simulink model "test_MPC_var2"  (R2025b)
settings: Solver=VariableStepAuto  StartTime=0.0  StopTime=20  RelTol=1e-3
undefined symbols (not defined in the file): imp_amp_d, imp_dur_d, stp_amp_u, stp_tim_u
libraries: cstblocks x4, mpclib x1
settings Model: Creator=USER  LastModifiedBy=francesco
settings SolverCC: AlgebraicLoopSolver=TrustRegion
settings DebuggingCC: AlgebraicLoopMsg=none  UnconnectedInputMsg=warning  UnconnectedLineMsg=warning
settings ModelReferenceCC: EnableRefExpFcnMdlSchedulingChecks=on
settings RTWCC: GPUComputeCapability=3.5  DLArmComputeVersion=19.05

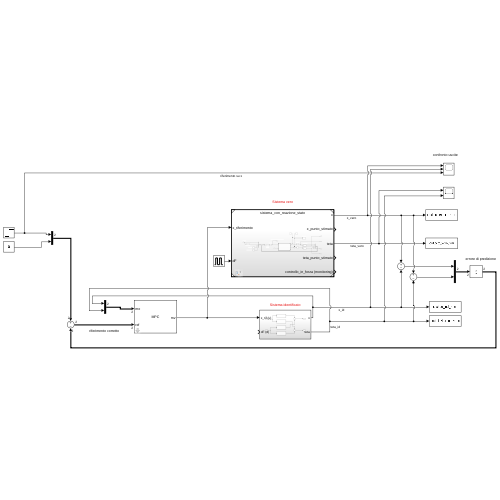
[thumbnail: Simulink's stored preview of the top-level diagram]
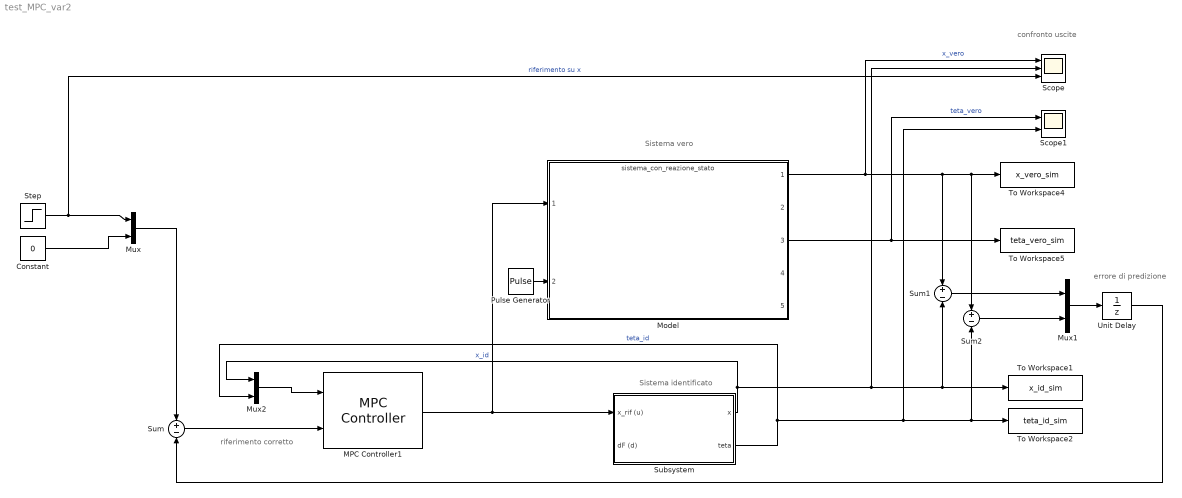
== system test_MPC_var2 ==
  note: riferimento corretto
  note: errore di predizione
  note: confronto uscite
  note: Sistema vero
  note: Sistema identificato
  Constant : Constant  Value=0
  MPC Controller1 : mpclib/MPC Controller  SCDEnableBlockLinearizationSpecification=on  mpcobj=mpc1  is_multiple=0  enable_value=0  return_u0=off  updateMPCinCallerWorkspace=on  md_inport=off  mv_inport=off  uref_inport=off  return_cost=off  return_mvseq=off  return_qpstatus=off  return_xseq=off  return_state=off  return_ovseq=off  state_inport=off  umin_inport=off  umax_inport=off  ymin_inport=off  ymax_inport=off  cc_inport=off  ywt_inport=off  uwt_inport=off  duwt_inport=off  rhoeps_inport=off  pm_inport=off  MaximumP=10  HorizonChoice=FixedHorizon  n_ts=0.2  n_p=10  n_mv=1  n_md=0  n_ud=1  n_mo=2  n_uo=0  BlockDataType=double  SampleTimeInherited=off  switch_inport=off
  Model : ModelReference  ModelNameDialog=sistema_con_reazione_stato.slx  SimulationMode=Normal  ModelReferenceVersion=9.56
  Mux : Mux  Inputs=2
  Mux1 : Mux  Inputs=2
  Mux2 : Mux  Inputs=2
  Pulse Generator : DiscretePulseGenerator  PulseType=Time based  Amplitude=imp_amp_d  Period=1000  PulseWidth=imp_dur_d / 1000 * 100  PhaseDelay=1
  Scope : Scope  NumInputPorts=3
      settings: ActiveDisplayYMinimum=-1.4761922699422587  ActiveDisplayYMaximum=11.58281196324811
  Scope1 : Scope  NumInputPorts=2
      settings: ActiveDisplayYMinimum=-0.74360512963747971  ActiveDisplayYMaximum=0.581453866823074
  Step : Step  Time=stp_tim_u  After=stp_amp_u  SampleTime=0
  Subsystem : Subsystem
  Sum : Sum  Inputs=+-
  Sum1 : Sum  Inputs=+-
  Sum2 : Sum  Inputs=+-
  To Workspace1 : ToWorkspace  VariableName=x_id_sim  SaveFormat=Timeseries  SampleTime=-1
  To Workspace2 : ToWorkspace  VariableName=teta_id_sim  SaveFormat=Timeseries  SampleTime=-1
  To Workspace4 : ToWorkspace  VariableName=x_vero_sim  SaveFormat=Timeseries  SampleTime=-1
  To Workspace5 : ToWorkspace  VariableName=teta_vero_sim  SaveFormat=Timeseries  SampleTime=-1
  Unit Delay : UnitDelay  SampleTime=-1  HasFrameUpgradeWarning=on
  wires:
  Model/1 -> Scope/1, Sum1/1, Sum2/1, To Workspace4/1  "x_vero"
  Model/3 -> Scope1/1, To Workspace5/1  "teta_vero"
  Subsystem/1(x) -> Mux2/1, Scope/2, Sum1/2, To Workspace1/1  "x_id"
  Subsystem/2(teta) -> Mux2/2, Scope1/2, Sum2/2, To Workspace2/1  "teta_id"
  Step/1 -> Mux/1, Scope/3  "riferimento su x"
  Constant/1 -> Mux/2
  MPC Controller1/1 -> Subsystem/1(x_rif (u)), Model/1
  Mux2/1 -> MPC Controller1/1
  Pulse Generator/1 -> Model/2
  Sum/1 -> MPC Controller1/2
  Sum2/1 -> Mux1/2
  Sum1/1 -> Mux1/1
  Mux/1 -> Sum/1
  Mux1/1 -> Unit Delay/1
  Unit Delay/1 -> Sum/2

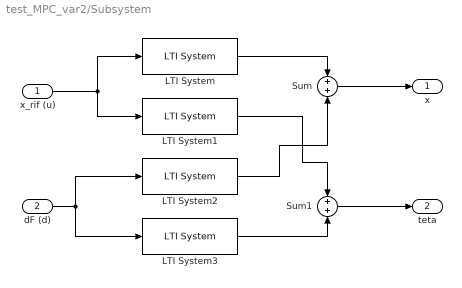
== system test_MPC_var2/Subsystem ==
  x_rif (u) : Inport
  dF (d) : Inport  Port=2
  LTI System : cstblocks/LTI System  sys=G_u_x  IC=[]  PadeOrder=0
  LTI System1 : cstblocks/LTI System  sys=G_u_teta  IC=[]  PadeOrder=0
  LTI System2 : cstblocks/LTI System  sys=G_d_x  IC=[]  PadeOrder=0
  LTI System3 : cstblocks/LTI System  sys=G_d_teta  IC=[]  PadeOrder=0
  Sum : Sum  Inputs=+|+
  Sum1 : Sum  Inputs=+|+
  x : Outport
  teta : Outport  Port=2
  wires:
  x_rif (u)/1 -> LTI System1/1, LTI System/1
  dF (d)/1 -> LTI System2/1, LTI System3/1
  LTI System/1 -> Sum/1
  Sum/1 -> x/1
  LTI System3/1 -> Sum1/2
  Sum1/1 -> teta/1
  LTI System2/1 -> Sum/2
  LTI System1/1 -> Sum1/1
